simulink model "Copy_9_of_SIMSCAPE_SIM_PROTOTYPE"  (R2024b)
settings: Solver=ode15s  StartTime=0.0  StopTime=T_sim  MaxStep=1e-6  RelTol=1e-6
InitFcn:
  | run param_file.m
values from neighbouring files (symbols this model uses):
  param = struct()    [Copy_of_param_file.m]    (also in param_file.m; param_file_loss_vs_freq.m; param_file_original.m; param_file_turbine.m)
libraries: fl_lib x49, nesl_utility x34, SimscapeFluids_lib x4, eeDcCurrentController x1, ee_lib x1
(part 1 of 2)
settings Model: Creator=user  LastModifiedBy=user
settings SolverCC: MaxConsecutiveMinStep=1000  ZeroCrossAlgorithm=Adaptive
settings DebuggingCC: AlgebraicLoopMsg=none  IgnoredZcDiagnostic=none

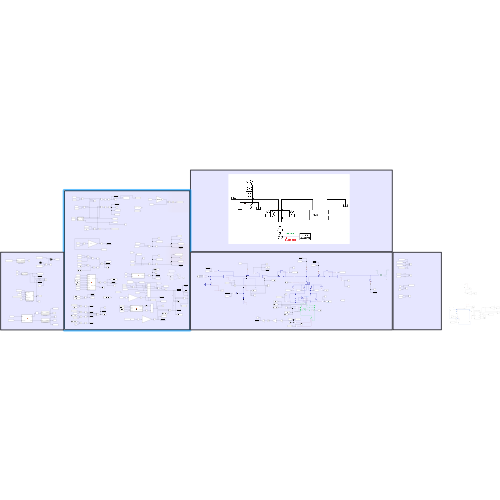
[thumbnail: Simulink's stored preview of the top-level diagram]
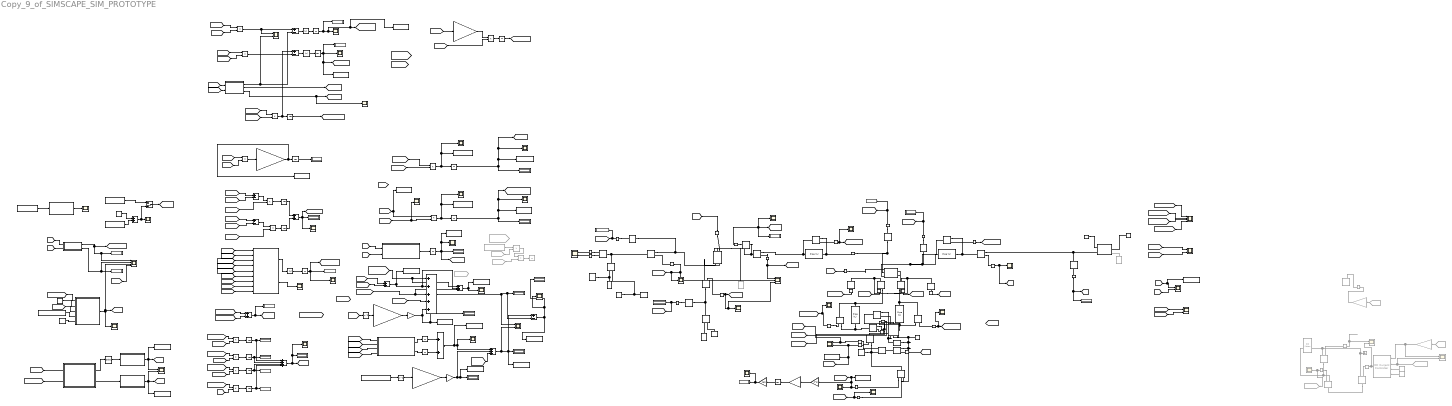
== system Copy_9_of_SIMSCAPE_SIM_PROTOTYPE ==
  note: Control
  note: Energy Calculations
  note: Circuit
  4-Way 2-Position Directional Valve (IL) : SimscapeFluids_lib/Isothermal Liquid/Valves & Orifices/Directional Control Valves/4-Way 2-Position Directional Valve (IL)  open_orifices_pos=fluids.isothermal_liquid.valves_orifices.directional_control_valves.enum.OpenOrifices4Way2Position.PA_BT  open_orifices_neg=fluids.isothermal_liquid.valves_orifices.directional_control_valves.enum.OpenOrifices4Way2Position.PB_AT  area_spec=fluids.isothermal_liquid.valves_orifices.directional_control_valves.enum.directional_valve_area_spec.identical  valve_spec=fluids.isothermal_liquid.valves_orifices.directional_control_valves.enum.directional_valve_spec.linear  del_S_max=param.stroke m  area_max=param.max_Avt m^2  del_S_TLU=[0, .00125, .0025, .00375, .005] m  valve_area_TLU=[1e-10, 1e-05, 4e-05, 6e-05, .0001] m^2  del_S_vol_flow_TLU=[0, .00125, .0025, .00375, .005] m  p_diff_TLU=[-.1, .3, .5, .7] MPa  vol_flow_TLU=[-1e-08, 2.2e-08, 2.8e-08, 3.4e-08; -9e-06, .00015, .0002, .00024; -.00036, .00063, .00081, .00096; -.00054, .00094, .0012, .0014; -.00091, .0016, .002, .0024] m^3/s  p_diff_TLU_const=[-.1, .3, .5, .7] MPa  vol_flow_TLU_const=[-.0009, .0016, .002, .0024] m^3/s  area_const=1e-4 m^2  area_leak=1e-10 m^2  area=inf m^2  Cd=0.64  Re_c=150  smoothing_factor=0.01  pressure_recovery=false  S_max_PA=5e-3 m  del_S_max_PA=0.005 m  area_max_PA=1e-4 m^2  del_S_TLU_PA=[0, .00125, .0025, .00375, .005] m  valve_area_TLU_PA=[1e-10, 1e-05, 4e-05, 6e-05, .0001] m^2  del_S_vol_flow_TLU_PA=[0, .00125, .0025, .00375, .005] m  p_diff_TLU_PA=[-.1, .3, .5, .7] MPa  vol_flow_TLU_PA=[-1e-08, 2.2e-08, 2.8e-08, 3.4e-08; -9e-06, .00015, .0002, .00024; -.00036, .00063, .00081, .00096; -.00054, .00094, .0012, .0014; -.00091, .0016, .002, .0024] m^3/s  area_const_PA=1e-4 m^2  p_diff_TLU_const_PA=[-.1, .3, .5, .7] MPa  vol_flow_TLU_const_PA=[-.0009, .0016, .002, .0024] m^3/s  S_max_PB=-5e-3 m  del_S_max_PB=0.005 m  area_max_PB=1e-4 m^2  del_S_TLU_PB=[0, .00125, .0025, .00375, .005] m  valve_area_TLU_PB=[1e-10, 1e-05, 4e-05, 6e-05, .0001] m^2  del_S_vol_flow_TLU_PB=[0, .00125, .0025, .00375, .005] m  p_diff_TLU_PB=[-.1, .3, .5, .7] MPa  vol_flow_TLU_PB=[-1e-08, 2.2e-08, 2.8e-08, 3.4e-08; -9e-06, .00015, .0002, .00024; -.00036, .00063, .00081, .00096; -.00054, .00094, .0012, .0014; -.00091, .0016, .002, .0024] m^3/s  area_const_PB=1e-4 m^2  p_diff_TLU_const_PB=[-.1, .3, .5, .7] MPa  vol_flow_TLU_const_PB=[-.0009, .0016, .002, .0024] m^3/s  S_max_AT=-5e-3 m  del_S_max_AT=0.005 m  area_max_AT=1e-4 m^2  del_S_TLU_AT=[0, .00125, .0025, .00375, .005] m  valve_area_TLU_AT=[1e-10, 1e-05, 4e-05, 6e-05, .0001] m^2  del_S_vol_flow_TLU_AT=[0, .00125, .0025, .00375, .005] m  p_diff_TLU_AT=[-.1, .3, .5, .7] MPa  vol_flow_TLU_AT=[-1e-08, 2.2e-08, 2.8e-08, 3.4e-08; -9e-06, .00015, .0002, .00024; -.00036, .00063, .00081, .00096; -.00054, .00094, .0012, .0014; -.00091, .0016, .002, .0024] m^3/s  area_const_AT=1e-4 m^2  p_diff_TLU_const_AT=[-.1, .3, .5, .7] MPa  vol_flow_TLU_const_AT=[-.0009, .0016, .002, .0024] m^3/s  S_max_BT=5e-3 m  del_S_max_BT=0.005 m  area_max_BT=1e-4 m^2  del_S_TLU_BT=[0, .00125, .0025, .00375, .005] m  valve_area_TLU_BT=[1e-10, 1e-05, 4e-05, 6e-05, .0001] m^2  del_S_vol_flow_TLU_BT=[0, .00125, .0025, .00375, .005] m  p_diff_TLU_BT=[-.1, .3, .5, .7] MPa  vol_flow_TLU_BT=[-1e-08, 2.2e-08, 2.8e-08, 3.4e-08; -9e-06, .00015, .0002, .00024; -.00036, .00063, .00081, .00096; -.00054, .00094, .0012, .0014; -.00091, .0016, .002, .0024] m^3/s  area_const_BT=1e-4 m^2  p_diff_TLU_const_BT=[-.1, .3, .5, .7] MPa  vol_flow_TLU_const_BT=[-.0009, .0016, .002, .0024] m^3/s
      settings: InternalSimscapePortConfiguration="{\"Bottom\":[{\"id\":\"P\",\"label\":\"P\",\"type\":\"foundation.isothermal_liquid.isothermal_liquid\"},{\"id\":\"T\",\"label\":\"T\",\"type\":\"foundation.isothermal_liquid.isothermal_liquid\"}],\"Left\":[{\"id\":\"S\",\"label\":\"S\",\"type\":\"input\"}],\"Right\":[],\"Top\":[{\"id\":\"A\",\"label\":\"A\",\"type\":\"foundation.isothermal_liquid.isothermal_liquid\"},{\"id\":\"B\",\"label\":\"B\",\"type\":\"foundation.isothermal_liquid.isothermal_liquid\"}]}"
  4-Way 3-Position Directional Valve (IL) : SimscapeFluids_lib/Isothermal Liquid/Valves & Orifices/Directional Control Valves/4-Way 3-Position Directional Valve (IL)  open_orifices_pos=fluids.isothermal_liquid.valves_orifices.directional_control_valves.enum.directional_valve_open_orifices_pos_neg.PA_BT  open_orifices_neu=fluids.isothermal_liquid.valves_orifices.directional_control_valves.enum.directional_valve_open_orifices_neutral.PA_PB_AT_BT  open_orifices_neg=fluids.isothermal_liquid.valves_orifices.directional_control_valves.enum.directional_valve_open_orifices_pos_neg.PB_AT  neutral_assert_action=simscape.enum.assert.action.warn  area_spec=fluids.isothermal_liquid.valves_orifices.directional_control_valves.enum.directional_valve_area_spec.identical  valve_spec=fluids.isothermal_liquid.valves_orifices.directional_control_valves.enum.directional_valve_spec.linear  del_S_max=param.stroke m  area_max=param.max_Avt m^2  del_S_TLU=[0, .00125, .0025, .00375, .005] m  valve_area_TLU=[1e-10, 1e-05, 4e-05, 6e-05, .0001] m^2  del_S_vol_flow_TLU=[0, .00125, .0025, .00375, .005] m  p_diff_TLU=[-.1, .3, .5, .7] MPa  vol_flow_TLU=[-1e-08, 2.2e-08, 2.8e-08, 3.4e-08; -9e-06, .00015, .0002, .00024; -.00036, .00063, .00081, .00096; -.00054, .00094, .0012, .0014; -.00091, .0016, .002, .0024] m^3/s  p_diff_TLU_const=[-.1, .3, .5, .7] MPa  vol_flow_TLU_const=[-.0009, .0016, .002, .0024] m^3/s  area_const=1e-4 m^2  area_leak=1e-10 m^2  area=inf m^2  Cd=0.64  Re_c=150  smoothing_factor=0.01  pressure_recovery=false  S_max_PA=2.5e-3 m  del_S_max_PA=0.005 m  area_max_PA=1e-4 m^2  del_S_TLU_PA=[0, .00125, .0025, .00375, .005] m  valve_area_TLU_PA=[1e-10, 1e-05, 4e-05, 6e-05, .0001] m^2  del_S_vol_flow_TLU_PA=[0, .00125, .0025, .00375, .005] m  p_diff_TLU_PA=[-.1, .3, .5, .7] MPa  vol_flow_TLU_PA=[-1e-08, 2.2e-08, 2.8e-08, 3.4e-08; -9e-06, .00015, .0002, .00024; -.00036, .00063, .00081, .00096; -.00054, .00094, .0012, .0014; -.00091, .0016, .002, .0024] m^3/s  area_const_PA=1e-4 m^2  p_diff_TLU_const_PA=[-.1, .3, .5, .7] MPa  vol_flow_TLU_const_PA=[-.0009, .0016, .002, .0024] m^3/s  S_max_PB=-2.5e-3 m  del_S_max_PB=0.005 m  area_max_PB=1e-4 m^2  del_S_TLU_PB=[0, .00125, .0025, .00375, .005] m  valve_area_TLU_PB=[1e-10, 1e-05, 4e-05, 6e-05, .0001] m^2  del_S_vol_flow_TLU_PB=[0, .00125, .0025, .00375, .005] m  p_diff_TLU_PB=[-.1, .3, .5, .7] MPa  vol_flow_TLU_PB=[-1e-08, 2.2e-08, 2.8e-08, 3.4e-08; -9e-06, .00015, .0002, .00024; -.00036, .00063, .00081, .00096; -.00054, .00094, .0012, .0014; -.00091, .0016, .002, .0024] m^3/s  area_const_PB=1e-4 m^2  p_diff_TLU_const_PB=[-.1, .3, .5, .7] MPa  vol_flow_TLU_const_PB=[-.0009, .0016, .002, .0024] m^3/s  S_max_AB=7.5e-3 m  del_S_max_AB=0.005 m  area_max_AB=1e-4 m^2  del_S_TLU_AB=[0, .00125, .0025, .00375, .005] m  valve_area_TLU_AB=[1e-10, 1e-05, 4e-05, 6e-05, .0001] m^2  del_S_vol_flow_TLU_AB=[0, .00125, .0025, .00375, .005] m  p_diff_TLU_AB=[-.1, .3, .5, .7] MPa  vol_flow_TLU_AB=[-1e-08, 2.2e-08, 2.8e-08, 3.4e-08; -9e-06, .00015, .0002, .00024; -.00036, .00063, .00081, .00096; -.00054, .00094, .0012, .0014; -.00091, .0016, .002, .0024] m^3/s  area_const_AB=1e-4 m^2  p_diff_TLU_const_AB=[-.1, .3, .5, .7] MPa  vol_flow_TLU_const_AB=[-.0009, .0016, .002, .0024] m^3/s  S_max_AT=-2.5e-3 m  del_S_max_AT=0.005 m  area_max_AT=1e-4 m^2  del_S_TLU_AT=[0, .00125, .0025, .00375, .005] m  valve_area_TLU_AT=[1e-10, 1e-05, 4e-05, 6e-05, .0001] m^2  del_S_vol_flow_TLU_AT=[0, .00125, .0025, .00375, .005] m  p_diff_TLU_AT=[-.1, .3, .5, .7] MPa  vol_flow_TLU_AT=[-1e-08, 2.2e-08, 2.8e-08, 3.4e-08; -9e-06, .00015, .0002, .00024; -.00036, .00063, .00081, .00096; -.00054, .00094, .0012, .0014; -.00091, .0016, .002, .0024] m^3/s  area_const_AT=1e-4 m^2  p_diff_TLU_const_AT=[-.1, .3, .5, .7] MPa  vol_flow_TLU_const_AT=[-.0009, .0016, .002, .0024] m^3/s  S_max_BT=2.5e-3 m  del_S_max_BT=0.005 m  area_max_BT=1e-4 m^2  del_S_TLU_BT=[0, .00125, .0025, .00375, .005] m  valve_area_TLU_BT=[1e-10, 1e-05, 4e-05, 6e-05, .0001] m^2  del_S_vol_flow_TLU_BT=[0, .00125, .0025, .00375, .005] m  p_diff_TLU_BT=[-.1, .3, .5, .7] MPa  vol_flow_TLU_BT=[-1e-08, 2.2e-08, 2.8e-08, 3.4e-08; -9e-06, .00015, .0002, .00024; -.00036, .00063, .00081, .00096; -.00054, .00094, .0012, .0014; -.00091, .0016, .002, .0024] m^3/s  area_const_BT=1e-4 m^2  p_diff_TLU_const_BT=[-.1, .3, .5, .7] MPa  vol_flow_TLU_const_BT=[-.0009, .0016, .002, .0024] m^3/s  S_max_PT=0 m  del_S_max_PT=0.005 m  area_max_PT=1e-4 m^2  del_S_TLU_PT=[0, .00125, .0025, .00375, .005] m  valve_area_TLU_PT=[1e-10, 1e-05, 4e-05, 6e-05, .0001] m^2  del_S_vol_flow_TLU_PT=[0, .00125, .0025, .00375, .005] m  p_diff_TLU_PT=[-.1, .3, .5, .7] MPa  vol_flow_TLU_PT=[-1e-08, 2.2e-08, 2.8e-08, 3.4e-08; -9e-06, .00015, .0002, .00024; -.00036, .00063, .00081, .00096; -.00054, .00094, .0012, .0014; -.00091, .0016, .002, .0024] m^3/s
      settings: InternalSimscapePortConfiguration="{\"Bottom\":[{\"id\":\"P\",\"label\":\"P\",\"type\":\"foundation.isothermal_liquid.isothermal_liquid\"},{\"id\":\"T\",\"label\":\"T\",\"type\":\"foundation.isothermal_liquid.isothermal_liquid\"}],\"Left\":[{\"id\":\"S\",\"label\":\"S\",\"type\":\"input\"}],\"Right\":[],\"Top\":[{\"id\":\"A\",\"label\":\"A\",\"type\":\"foundation.isothermal_liquid.isothermal_liquid\"},{\"id\":\"B\",\"label\":\"B\",\"type\":\"foundation.isothermal_liquid.isothermal_liquid\"}]}"
  Abs : Abs  SaturateOnIntegerOverflow=off
  Abs1 : Abs  SaturateOnIntegerOverflow=off
  Abs2 : Abs  SaturateOnIntegerOverflow=off
  Add : Sum  Inputs=+++++
  Add1 : Sum  Inputs=+++
  Add{2..4,6..7} (5 alike) : Sum
  Add5 : Sum  Inputs=++++
  Add8 : Sum  Inputs=+++
  Constant : Constant  Value=param.stroke
  Constant1 : Constant  Value=param.start_final_velocity
  Constant2 : Constant  Value=param.P_H
  Constant3 : Constant  Value=0.75
  Constant4 : Constant  Value=15
  Constant5 : Constant  Value=param.start_final_velocity
  Constant6 : Constant  Value=param.P_M
  Constant7 : Constant  Commented=on  Value=24
  Constant8 : Constant  Commented=on  Value=0
  Constant9 : Constant  Commented=on  Value=param.damping
  Controlled Current Source : fl_lib/Electrical/Electrical Sources/Controlled Current Source  Commented=on
  Controlled Voltage Source : fl_lib/Electrical/Electrical Sources/Controlled Voltage Source  Commented=on
  Current Sensor : fl_lib/Electrical/Electrical Sensors/Current Sensor  Commented=on
  DC Current Controller : eeDcCurrentController/DC Current Controller  Commented=on  Kp=10  Ki=5  Kaw=1  VoltLim=Positive and negative voltage  Ts=-1  Tsd=0.001  ActZC=off
      settings: LibrarySourceBlock=|
      | ee_sl_lib/General Machine
      | Control/DC Current Controller
  DC Motor : ee_lib/Electromechanical/Brushed Motors/DC Motor  Commented=on  field_option=ee.enum.field_option.pm  Rf=100 Ohm  Lf=1 H  Laf=0.15 H  If0=0 A  parameterization=ee.enum.dcparam_option.load_speed  Ra=0.522 Ohm  La=0.625 mH  emf_or_torque=ee.enum.emf_or_torque.ki  Kv=1/param.Kv V*s/rad  Ki=param.Kt N*m/A  T_stall=7480 m*mN  w_max=3120 rpm  w_rated=2510 rpm  P_rated=147 W  V_rated=36 V  lam_param=ee.enum.lam_param.current  i_noload=348 mA  V_i_noload=36 V  J=0 kg*m^2  lam=0 N*m*s/rad  speed0=param.start_final_velocity rad/s  t_fault_armature=1 s  t_fault_field=1 s  fault_action=simscape.enum.assert.action.none  alpha=3.93e-3 1/K  Tmeas=25 degC  thermal_mass=100 J/K  initial_temperature=25 degC
  Display{,1..16} (17 alike) : Display
  Double-Acting Actuator (IL)1 : SimscapeFluids_lib/Isothermal Liquid/Actuators/Double-Acting Actuator (IL)  single_fluid=true  mech_orientation=foundation.enum.MechOrientationTranslational.Positive  piston_area_A=param.Acap m^2  piston_area_B=4e-4 m^2  stroke=param.V1_0/param.Acap m  dead_volume_A=1e-5 m^3  dead_volume_B=1e-5 m^3  pressure_spec=foundation.enum.pressure_spec.atmospheric  environment_pressure=0.101325 MPa  hardstop_model=simscape.enum.hardstop.smooth  stiff_coeff=1e10 N/m  damping_coeff=150 N*s/m  transition=0.1 mm  coeff_rest=0.7  v_tol=0.001 m/s  f_tol=0.001 N  cushion_A_spec=false  area_plunger_A=1e-4 m^2  length_plunger_A=1e-3 m  area_cushion_orifice_A=1e-6 m^2  area_leak_plunger_A=1e-7 m^2  p_crack_differential_A=0.01 MPa  press_max_differential_A=0.1 MPa  check_valve_area_max_A=1e-4 m^2  check_valve_area_leak_A=1e-10 m^2  smoothing_factor_A=0.01  cushion_B_spec=false  area_plunger_B=1e-4 m^2  length_plunger_B=1e-3 m  area_cushion_orifice_B=1e-6 m^2  area_leak_plunger_B=1e-7 m^2  p_crack_differential_B=0.01 MPa  press_max_differential_B=0.1 MPa  check_valve_area_max_B=1e-4 m^2  check_valve_area_leak_B=1e-10 m^2  smoothing_factor_B=0.01  friction_spec=false  breakaway_Coulomb_ratio=1.2  breakaway_velocity=0.1 m/s  preload_force=20 N  Coulomb_coeff=1e-6 N/Pa  viscous_coeff=100 N*s/m  leakage_spec=false  clearance=1e-4 m  piston_length=0.01 m  displacement_spec=foundation.enum.DisplacementSpec.Calculate  x0=param.V1_0/param.Acap m  dynamic_compressibility=true  p0_A=param.P_initial+param.P_T Pa  p0_B=param.P_T Pa
      settings: InternalSimscapePortConfiguration="{\"Bottom\":[],\"Left\":[{\"id\":\"C\",\"label\":\"C\",\"type\":\"foundation.mechanical.translational.translational\"},{\"id\":\"A\",\"label\":\"A\",\"type\":\"foundation.isothermal_liquid.isothermal_liquid\"}],\"Right\":[{\"id\":\"p_out\",\"label\":\"p\",\"type\":\"output\"},{\"id\":\"R\",\"label\":\"R\",\"type\":\"foundation.mechanical.translational.translational\"},{\"id\":\"B\",\"label\":\"B\",\"type\":\"foundation.isothermal_liquid.isothermal_liquid\"}],\"Top\":[]}"
  Dynamics of Orifice 3 : Subsystem
  Electric Torque Controller1 : MATLAB Function  TreatAsAtomicUnit=on
  Electrical Reference : fl_lib/Electrical/Electrical Elements/Electrical Reference  Commented=on
  Energy In : Display
  Energy Out : Display
  Fixed-Displacement Motor (IL) : SimscapeFluids_lib/Isothermal Liquid/Pumps & Motors/Fixed-Displacement Motor (IL)  leakage_friction_spec=fluids.isothermal_liquid.pumps_motors.enum.MotorLossSpec.Analytical  displacement=param.D m^3/rev  omega_nominal=1000 rpm  p_nominal=21 MPa  vol_eff_nominal=param.pump_vol_eff  mech_eff_nominal=param.pump_mech_eff  no_load_torque=0 N*m  p_diff_eff_TLU=[.1, 1, 2] MPa  omega_eff_TLU=[250, 500, 1000, 2000, 3000, 4000] rpm  vol_eff_TLU=[.816, .908, .954, .977, .981, .984; .325, .663, .831, .916, .925, .946; .137, .568, .78, .892, .893, .91]  mech_eff_TLU=[.996, .996, .996, .996, .996, .996; .988, .989, .989, .989, .989, .99; .981, .981, .982, .982, .983, .984]  p_diff_loss_TLU=[.1, 1, 2] MPa  omega_loss_TLU=[250, 500, 1000, 2000, 3000, 4000] rpm  vol_loss_TLU=1e-3 * [.023, .023, .023, .023, .0285, .032; .0844, .0842, .0845, .084, .1125, .108; .1079, .108, .11, .108, .1605, .18] m^3/s  mech_loss_TLU=[.002, .002, .002, .002, .002, .002; .0607, .0556, .0556, .0556, .0556, .0505; .1937, .1937, .1833, .1833, .1729, .1626] N*m  q_shaft_TLU=[.125, .25, .5, 1, 1.5, 2] * 1e-3 m^3/s  p_diff_shaft_TLU=[.1, 1, 2] MPa  torque_shaft_TLU=[.47, 4.72, 9.35; .47, 4.7, 9.36; .47, 4.7, 9.4; .47, 4.7, 9.41; .47, 4.7, 9.46; .47, 4.68, 9.5] N*m  omega_shaft_TLU=[205, 80, 35; 455, 330, 285; 955, 831, 780; 1950, 1830, 1780; 2940, 2775, 2680; 3940, 3780, 3640] rpm  vol_eff_min=1e-3  vol_eff_max=1  mech_eff_min=1e-3  mech_eff_max=1  pressure_threshold=1e-3 MPa  omega_threshold=100 rpm  supplied_range_check=simscape.enum.assert.action.none  motor_mode_check=simscape.enum.assert.action.none  pressure_check=simscape.enum.assert.action.none  p_min_valid=0.101325 MPa
      settings: InternalSimscapePortConfiguration="{\"Bottom\":[{\"id\":\"B\",\"label\":\"B\",\"type\":\"foundation.isothermal_liquid.isothermal_liquid\"}],\"Left\":[],\"Right\":[{\"id\":\"R\",\"label\":\"R\",\"type\":\"foundation.mechanical.rotational.rotational\"},{\"id\":\"C\",\"label\":\"C\",\"type\":\"foundation.mechanical.rotational.rotational\"}],\"Top\":[{\"id\":\"A\",\"label\":\"A\",\"type\":\"foundation.isothermal_liquid.isothermal_liquid\"}]}"
  Flow Rate Sensor (IL){,1..7} (8 alike) : fl_lib/Isothermal Liquid/Sensors/Flow Rate Sensor (IL)  sensor_type=foundation.enum.mass_volumetric_sensor.volumetric
      settings: InternalSimscapePortConfiguration="{\"Bottom\":[],\"Left\":[{\"id\":\"A\",\"label\":\"A\",\"type\":\"foundation.isothermal_liquid.isothermal_liquid\"}],\"Right\":[{\"id\":\"B\",\"label\":\"B\",\"type\":\"foundation.isothermal_liquid.isothermal_liquid\"},{\"id\":\"V\",\"label\":\"V\",\"type\":\"output\"}],\"Top\":[]}"
  For the big Valve : Subsystem
  For the small Valve : Subsystem
  From11 : From  Commented=on  GotoTag=T_elec
  From46 : From  Commented=on  GotoTag=Current_arm
  From54 : From  Commented=on  GotoTag=T_elec
  From62 : From  Commented=on  GotoTag=omega
  From63 : From  Commented=on  GotoTag=omega
  From77 : From  Commented=on  GotoTag=elec_motor_losses
  From79 : From  Commented=on  GotoTag=Regen_Elec
  Gain : Gain  Commented=on  Gain=1/(param.Kt)
  Gain1 : Gain  Gain=param.J_elec+param.J_hyd
  Gain10 : Gain  Gain=param.damping
  Gain2 : Gain  Gain=0.5
  Gain3 : Gain  Gain=param.D
  Gain4 : Gain  Gain=param.J_elec+param.J_hyd
  Gain5 : Gain  Gain=0.5
  Gain6 : Gain  Gain=param.J_elec+param.J_hyd
  Gain7 : Gain  Commented=on  Gain=1/(param.Kt)
  Gain8 : Gain  Gain=2*pi
  Gain9 : Gain  Gain=1e6
  Goto30 : Goto  Commented=on  GotoTag=Current_arm
  Hydraulic Motor Inertia : fl_lib/Mechanical/Rotational Elements/Inertia  inertia=(param.J_hyd+param.J_elec) kg*m^2  num_ports=foundation.enum.numPorts2.one  w_specify=on  w_priority=High  w=param.start_final_velocity rad/s  w_nominal_specify=off  w_nominal_value=1  w_nominal_unit=rad/s  t_specify=off  t_priority=None  t=0 N*m  t_nominal_specify=off  t_nominal_value=1  t_nominal_unit=N*m
  Ideal Rotational Motion Sensor1 : fl_lib/Mechanical/Mechanical Sensors/Ideal Rotational Motion Sensor  reference=foundation.enum.MeasurementReference.difference  acceleration_port=true  velocity_port=true  position_port=false  wrap_angle=false  offset=0 rad
      settings: InternalSimscapePortConfiguration="{\"Bottom\":[],\"Left\":[{\"id\":\"R\",\"label\":\"R\",\"type\":\"foundation.mechanical.rotational.rotational\"}],\"Right\":[{\"id\":\"C\",\"label\":\"C\",\"type\":\"foundation.mechanical.rotational.rotational\"},{\"id\":\"alpha\",\"label\":\"α\",\"type\":\"output\"},{\"id\":\"W\",\"label\":\"W\",\"type\":\"output\"}],\"Top\":[]}"
  Ideal Torque Sensor : fl_lib/Mechanical/Mechanical Sensors/Ideal Torque Sensor
  Ideal Torque Sensor1 : fl_lib/Mechanical/Mechanical Sensors/Ideal Torque Sensor
  Ideal Torque Source : fl_lib/Mechanical/Mechanical Sources/Ideal Torque Source
  Initial Kinetic Energy : Display
  Integrator{,1..10,12,14..17,20..21} (18 alike) : Integrator
  Integrator13 : Integrator  Commented=on
  Isothermal Liquid Properties (IL) : fl_lib/Isothermal Liquid/Utilities/Isothermal Liquid Properties (IL)  rho_L_atm=param.rho kg/m^3  bulk_modulus_model=foundation.enum.bulk_modulus_model.const  beta_gain=6  beta_L_atm=param.beta Pa  nu_atm=1.0034e-6 m^2/s  p_atm=0.101325 MPa  p_min=1 Pa  properties_range_check=simscape.enum.assert.action.error  air_fraction=0.005  polytropic_index=1.0  rho_g_atm=1.225 kg/m^3  air_dissolution_model=false  p_crit=1 MPa
  Liquid Properties Sensor (IL) : fl_lib/Isothermal Liquid/Sensors/Liquid Properties Sensor (IL)  density_measure=false  bulk_modulus_measure=true  entrained_air_measure=true
      settings: InternalSimscapePortConfiguration="{\"Bottom\":[],\"Left\":[{\"id\":\"A\",\"label\":\"A\",\"type\":\"foundation.isothermal_liquid.isothermal_liquid\"}],\"Right\":[{\"id\":\"beta\",\"label\":\"beta\",\"type\":\"output\"},{\"id\":\"theta\",\"label\":\"theta\",\"type\":\"output\"}],\"Top\":[]}"
  MATLAB Function1 : MATLAB Function  TreatAsAtomicUnit=on
  MATLAB Function2 : MATLAB Function  TreatAsAtomicUnit=on
  MATLAB Function3 : MATLAB Function  TreatAsAtomicUnit=on
  MATLAB Function4 : MATLAB Function  TreatAsAtomicUnit=on
  MATLAB Function6 : MATLAB Function  TreatAsAtomicUnit=on
  Manual Switch : ManualSwitch  CurrentSetting=0
  Mechanical Rotational Reference2 : fl_lib/Mechanical/Rotational Elements/Mechanical Rotational Reference
  Mechanical Translational Reference2 : fl_lib/Mechanical/Translational Elements/Mechanical Translational Reference
  Mechanical Translational Reference3 : fl_lib/Mechanical/Translational Elements/Mechanical Translational Reference
  Mechanical Energy : Display
  PS Constant : fl_lib/Physical Signals/Sources/PS Constant  constant=param.P_H Pa
  PS Constant1 : fl_lib/Physical Signals/Sources/PS Constant  constant=param.P_M Pa
  PS-Simulink Converter : nesl_utility/PS-Simulink Converter  PhysicalDomain=network_engine_domain  SubClassName=ps_output  LeftPortType=input  RightPortType=output  PseudoPeriodic=off  Frequencies=[]  VectorFormat=inherit  Unit=m^3/s  AffineConversion=off
  PS-Simulink Converter1 : nesl_utility/PS-Simulink Converter  PhysicalDomain=network_engine_domain  SubClassName=ps_output  LeftPortType=input  RightPortType=output  PseudoPeriodic=off  Frequencies=[]  VectorFormat=inherit  Unit=rad/s  AffineConversion=off
  PS-Simulink Converter10 : nesl_utility/PS-Simulink Converter  PhysicalDomain=network_engine_domain  SubClassName=ps_output  LeftPortType=input  RightPortType=output  PseudoPeriodic=off  Frequencies=[]  VectorFormat=inherit  Unit=Pa  AffineConversion=off
  PS-Simulink Converter11 : nesl_utility/PS-Simulink Converter  PhysicalDomain=network_engine_domain  SubClassName=ps_output  LeftPortType=input  RightPortType=output  PseudoPeriodic=off  Frequencies=[]  VectorFormat=inherit  Unit=m^3/s  AffineConversion=off
  PS-Simulink Converter12 : nesl_utility/PS-Simulink Converter  PhysicalDomain=network_engine_domain  SubClassName=ps_output  LeftPortType=input  RightPortType=output  PseudoPeriodic=off  Frequencies=[]  VectorFormat=inherit  Unit=m^3/s  AffineConversion=off
  PS-Simulink Converter{3..9,13..19,21,23..27} (20 alike) : nesl_utility/PS-Simulink Converter  PhysicalDomain=network_engine_domain  SubClassName=ps_output  LeftPortType=input  RightPortType=output  PseudoPeriodic=off  Frequencies=[]  VectorFormat=inherit  Unit=inherit  AffineConversion=off
  PS-Simulink Converter2 : nesl_utility/PS-Simulink Converter  PhysicalDomain=network_engine_domain  SubClassName=ps_output  LeftPortType=input  RightPortType=output  PseudoPeriodic=off  Frequencies=[]  VectorFormat=inherit  Unit=Pa  AffineConversion=off
  PS-Simulink Converter20 : nesl_utility/PS-Simulink Converter  Commented=on  PhysicalDomain=network_engine_domain  SubClassName=ps_output  LeftPortType=input  RightPortType=output  PseudoPeriodic=off  Frequencies=[]  VectorFormat=inherit  Unit=inherit  AffineConversion=off
  PS-Simulink Converter22 : nesl_utility/PS-Simulink Converter  Commented=on  PhysicalDomain=network_engine_domain  SubClassName=ps_output  LeftPortType=input  RightPortType=output  PseudoPeriodic=off  Frequencies=[]  VectorFormat=inherit  Unit=inherit  AffineConversion=off
  Pipe (IL)2 : fl_lib/Isothermal Liquid/Elements/Pipe (IL)  length=0.2 m  area=0.25*pi*(param.D_hose)^2 mm^2  Dh=param.D_hose mm  length_add=0.5 m  roughness=15e-6 m  Re_lam=2000  Re_tur=4000  shape_factor=64  dynamic_compressibility=true  inertia=false  p0=param.P_initial+param.P_T Pa  mdot0=0 kg/s
      settings: InternalSimscapePortConfiguration="{\"Bottom\":[],\"Left\":[{\"id\":\"A\",\"label\":\"A\",\"type\":\"foundation.isothermal_liquid.isothermal_liquid\"}],\"Right\":[{\"id\":\"B\",\"label\":\"B\",\"type\":\"foundation.isothermal_liquid.isothermal_liquid\"}],\"Top\":[]}"
  Pipe (IL)3 : fl_lib/Isothermal Liquid/Elements/Pipe (IL)  length=0.2 m  area=0.25*pi*(param.D_hose)^2 mm^2  Dh=param.D_hose mm  length_add=0.5 m  roughness=15e-6 m  Re_lam=2000  Re_tur=4000  shape_factor=64  dynamic_compressibility=true  inertia=false  p0=param.P_initial+param.P_T Pa  mdot0=0 kg/s
      settings: InternalSimscapePortConfiguration="{\"Bottom\":[],\"Left\":[{\"id\":\"A\",\"label\":\"A\",\"type\":\"foundation.isothermal_liquid.isothermal_liquid\"}],\"Right\":[{\"id\":\"B\",\"label\":\"B\",\"type\":\"foundation.isothermal_liquid.isothermal_liquid\"}],\"Top\":[]}"
  Pipe (IL)4 : fl_lib/Isothermal Liquid/Elements/Pipe (IL)  length=0.2 m  area=0.25*pi*(param.D_hose)^2 mm^2  Dh=param.D_hose mm  length_add=0.5 m  roughness=15e-6 m  Re_lam=2000  Re_tur=4000  shape_factor=64  dynamic_compressibility=true  inertia=false  p0=param.P_initial+param.P_T Pa  mdot0=0 kg/s
      settings: InternalSimscapePortConfiguration="{\"Bottom\":[],\"Left\":[{\"id\":\"A\",\"label\":\"A\",\"type\":\"foundation.isothermal_liquid.isothermal_liquid\"}],\"Right\":[{\"id\":\"B\",\"label\":\"B\",\"type\":\"foundation.isothermal_liquid.isothermal_liquid\"}],\"Top\":[]}"
  Pipe (IL)5 : fl_lib/Isothermal Liquid/Elements/Pipe (IL)  length=1 m  area=0.25*pi*(param.D_hose)^2 mm^2  Dh=param.D_hose mm  length_add=0.5 m  roughness=15e-6 m  Re_lam=2000  Re_tur=4000  shape_factor=64  dynamic_compressibility=true  inertia=false  p0=param.P_initial+param.P_T Pa  mdot0=0 kg/s
      settings: InternalSimscapePortConfiguration="{\"Bottom\":[],\"Left\":[{\"id\":\"A\",\"label\":\"A\",\"type\":\"foundation.isothermal_liquid.isothermal_liquid\"}],\"Right\":[{\"id\":\"B\",\"label\":\"B\",\"type\":\"foundation.isothermal_liquid.isothermal_liquid\"}],\"Top\":[]}"
  Pressure Sensor (IL){,1..5,10..11} (8 alike) : fl_lib/Isothermal Liquid/Sensors/Pressure Sensor (IL)  pressure_measure=foundation.enum.pressure_measure.gauge
      settings: InternalSimscapePortConfiguration="{\"Bottom\":[],\"Left\":[{\"id\":\"A\",\"label\":\"A\",\"type\":\"foundation.isothermal_liquid.isothermal_liquid\"}],\"Right\":[{\"id\":\"Pg\",\"label\":\"Pg\",\"type\":\"output\"}],\"Top\":[]}"
  Pressure Sensor (IL){6..9,12} (5 alike) : fl_lib/Isothermal Liquid/Sensors/Pressure Sensor (IL)  pressure_measure=foundation.enum.pressure_measure.difference
      settings: InternalSimscapePortConfiguration="{\"Bottom\":[],\"Left\":[{\"id\":\"A\",\"label\":\"A\",\"type\":\"foundation.isothermal_liquid.isothermal_liquid\"}],\"Right\":[{\"id\":\"B\",\"label\":\"B\",\"type\":\"foundation.isothermal_liquid.isothermal_liquid\"},{\"id\":\"P\",\"label\":\"P\",\"type\":\"output\"}],\"Top\":[]}"
  Pressure Source (IL)1 : fl_lib/Isothermal Liquid/Sources/Pressure Source (IL)  source_type=foundation.enum.constant_controlled.controlled  pressure_differential=0 MPa
      settings: InternalSimscapePortConfiguration="{\"Bottom\":[],\"Left\":[{\"id\":\"A\",\"label\":\"A\",\"type\":\"foundation.isothermal_liquid.isothermal_liquid\"},{\"id\":\"P\",\"label\":\"P\",\"type\":\"input\"}],\"Right\":[{\"id\":\"B\",\"label\":\"B\",\"type\":\"foundation.isothermal_liquid.isothermal_liquid\"}],\"Top\":[]}"
  Pressure Source (IL)2 : fl_lib/Isothermal Liquid/Sources/Pressure Source (IL)  source_type=foundation.enum.constant_controlled.controlled  pressure_differential=0 MPa
      settings: InternalSimscapePortConfiguration="{\"Bottom\":[],\"Left\":[{\"id\":\"A\",\"label\":\"A\",\"type\":\"foundation.isothermal_liquid.isothermal_liquid\"},{\"id\":\"P\",\"label\":\"P\",\"type\":\"input\"}],\"Right\":[{\"id\":\"B\",\"label\":\"B\",\"type\":\"foundation.isothermal_liquid.isothermal_liquid\"}],\"Top\":[]}"
  Product{,1..10,13..14} (13 alike) : Product
  Product11 : Product  Commented=on
  Product12 : Product  Commented=on
  Pulse Generator : DiscretePulseGenerator  PulseType=Time based  Amplitude=param.P_H-param.P_M  Period=param.T_period  PulseWidth=50  PhaseDelay=param.delay
  Regen : Display
  Regen1 : Display
  Reservoir (IL)1 : fl_lib/Isothermal Liquid/Elements/Reservoir (IL)  reservoir_type=foundation.enum.constant_controlled.constant  pressure_spec=foundation.enum.pressure_spec.atmospheric  reservoir_pressure=0.101325 MPa
  Reservoir (IL)5 : fl_lib/Isothermal Liquid/Elements/Reservoir (IL)  reservoir_type=foundation.enum.constant_controlled.constant  pressure_spec=foundation.enum.pressure_spec.atmospheric  reservoir_pressure=0.101325 MPa
  Reservoir (IL)7 : fl_lib/Isothermal Liquid/Elements/Reservoir (IL)  Commented=on  reservoir_type=foundation.enum.constant_controlled.constant  pressure_spec=foundation.enum.pressure_spec.atmospheric  reservoir_pressure=0.101325 MPa
  Reservoir (IL)8 : fl_lib/Isothermal Liquid/Elements/Reservoir (IL)  Commented=on  reservoir_type=foundation.enum.constant_controlled.constant  pressure_spec=foundation.enum.pressure_spec.atmospheric  reservoir_pressure=0.101325 MPa
  Rotational Damper : fl_lib/Mechanical/Rotational Elements/Rotational Damper  D=param.damping N*m*s/rad  w_specify=on  w_priority=None  w=param.start_final_velocity rad/s  w_nominal_specify=off  w_nominal_value=1  w_nominal_unit=rad/s  t_specify=off  t_priority=None  t=0 N*m  t_nominal_specify=off  t_nominal_value=1  t_nominal_unit=N*m
  Scope{,1,4,6,8,16,23,27,41} (9 alike) : Scope  NumInputPorts=2
  Scope{2..3,7,10..15,17..21,26,28..34,36..40,42} (28 alike) : Scope
  Scope22 : Scope  Commented=on
  Scope24 : Scope  Commented=on  NumInputPorts=2
  Scope25 : Scope  Commented=on  NumInputPorts=2
  Scope35 : Scope  NumInputPorts=3
  Scope5 : Scope  NumInputPorts=4
  Scope9 : Scope  NumInputPorts=4
  Simulink-PS Converter : nesl_utility/Simulink-PS Converter  PhysicalDomain=network_engine_domain  SubClassName=ps_input  LeftPortType=input  RightPortType=output  PseudoPeriodic=off  Frequencies=[]  NoiseDistribution=none  NoiseParameters=[]  Unit=1  AffineConversion=off  FilteringAndDerivatives=provide  SimscapeFilterOrder=1  InputFilterTimeConstant=0.001  UdotUserProvided=0
  Simulink-PS Converter1 : nesl_utility/Simulink-PS Converter  PhysicalDomain=network_engine_domain  SubClassName=ps_input  LeftPortType=input  RightPortType=output  PseudoPeriodic=off  Frequencies=[]  NoiseDistribution=none  NoiseParameters=[]  Unit=1  AffineConversion=off  FilteringAndDerivatives=provide  SimscapeFilterOrder=1  InputFilterTimeConstant=0.001  UdotUserProvided=0
  Simulink-PS Converter2 : nesl_utility/Simulink-PS Converter  Commented=on  PhysicalDomain=network_engine_domain  SubClassName=ps_input  LeftPortType=input  RightPortType=output  PseudoPeriodic=off  Frequencies=[]  NoiseDistribution=none  NoiseParameters=[]  Unit=1  AffineConversion=off  FilteringAndDerivatives=provide  SimscapeFilterOrder=1  InputFilterTimeConstant=0.001  UdotUserProvided=0
  Simulink-PS Converter3 : nesl_utility/Simulink-PS Converter  Commented=on  PhysicalDomain=network_engine_domain  SubClassName=ps_input  LeftPortType=input  RightPortType=output  PseudoPeriodic=off  Frequencies=[]  NoiseDistribution=none  NoiseParameters=[]  Unit=1  AffineConversion=off  FilteringAndDerivatives=provide  SimscapeFilterOrder=1  InputFilterTimeConstant=0.001  UdotUserProvided=0
  Simulink-PS Converter4 : nesl_utility/Simulink-PS Converter  PhysicalDomain=network_engine_domain  SubClassName=ps_input  LeftPortType=input  RightPortType=output  PseudoPeriodic=off  Frequencies=[]  NoiseDistribution=none  NoiseParameters=[]  Unit=1  AffineConversion=off  FilteringAndDerivatives=provide  SimscapeFilterOrder=1  InputFilterTimeConstant=0.001  UdotUserProvided=0
  Solver Configuration1 : nesl_utility/Solver Configuration  PhysicalDomain=network_engine_domain  SubClassName=solver  LeftPortType=input  RightPortType=generic  Tones=[]  Harmonics=[]  SimulateNoise=off  Profile=off  UseLocalSampling=off  EnableSwitchedLinearOptims=on  FrequencyDomain=off  UseCCode=off  RelTol=0.001  AbsTol=0.001  MinStep=1e-09  ToWorkspace=off  RevertToSquareIcSolve=off  NumHomotopyIterations=100  PhasorMode=off  PhasorModeNumHarmonics=1  ConsistencySolver=NEWTON_XTOL_AFTER_FTOL  IndexReductionMethod=DerivativeReplacement  DoDC=off  ResidualTolerance=1e-09  ConsistencyTolSource=GLOBAL  ConsistencyAbsTol=0.001  ConsistencyRelTol=0.001  ConsistencyTolFactor=0.001  UseLocalSolver=off  LocalSolverChoice=NE_BACKWARD_EULER_ADVANCER  ResolveIndetEquations=on  FunctionEvalNumThread=1  LocalSolverSampleTime=0.001  DoFixedCost=off  MaxNonlinIter=3  MaxModeIter=2  ComputeImpulses=off  ImpulseIterations=2  LinearAlgebra=auto  LinearAlgebraNumThread=0  EquationFormulation=NE_TIME_EF  DelaysMemoryBudget=1024  AutomaticFiltering=on  FilteringTimeConstant=0.001  PartitionStorageMethod=AS_NEEDED  PartitionMemoryBudget=1024  PartitionMethod=ROBUST  MultibodyUseLocalSolver=off  MultibodyLocalSolverChoice=ODE1  MultibodyLocalSolverSampleTime=0.001
  Square1 : Math  Operator=square
  Square2 : Math  Operator=square
  Stored : Display
  Subsystem : Subsystem
  Subtract{,1..4} (5 alike) : Sum  Inputs=+-
  Throttling Loss Big Valve : Display
  Throttling Loss Small Valve1 : Display
  Throttling Total : Display
  To Workspace : ToWorkspace  VariableName=Stored  SaveFormat=Timeseries  SampleTime=-1
  To Workspace1 : ToWorkspace  VariableName=Regen_Mech  SaveFormat=Timeseries  SampleTime=-1
  To Workspace10 : ToWorkspace  VariableName=Hyd_Energy_In  SaveFormat=Timeseries  SampleTime=-1
  To Workspace11 : ToWorkspace  VariableName=Work_Out  SaveFormat=Timeseries  SampleTime=-1
  To Workspace12 : ToWorkspace  VariableName=Regen_Elec  SaveFormat=Timeseries  SampleTime=-1
  To Workspace13 : ToWorkspace  VariableName=Regen_power_Elec  SaveFormat=Timeseries  SampleTime=-1
  To Workspace14 : ToWorkspace  VariableName=Throttling_Losses  SaveFormat=Timeseries  SampleTime=-1
  To Workspace15 : ToWorkspace  VariableName=T_elec_2  SaveFormat=Timeseries  SampleTime=-1
  To Workspace16 : ToWorkspace  VariableName=Pump_Losses  SaveFormat=Timeseries  SampleTime=-1
  To Workspace17 : ToWorkspace  VariableName=elec_motor_losses  SaveFormat=Timeseries  SampleTime=-1
  To Workspace18 : ToWorkspace  VariableName=S_big  SaveFormat=Timeseries  SampleTime=-1
  To Workspace19 : ToWorkspace  VariableName=S_small  SaveFormat=Timeseries  SampleTime=-1
  To Workspace2 : ToWorkspace  VariableName=KE  SaveFormat=Timeseries  SampleTime=-1
  To Workspace20 : ToWorkspace  VariableName=Losses  SaveFormat=Timeseries  SampleTime=-1
  To Workspace3 : ToWorkspace  VariableName=P1  SaveFormat=Timeseries  SampleTime=-1
  To Workspace4 : ToWorkspace  VariableName=T_elec  SaveFormat=Timeseries  SampleTime=-1
  To Workspace5 : ToWorkspace  VariableName=omega  SaveFormat=Timeseries  SampleTime=-1
  To Workspace6 : ToWorkspace  VariableName=Regen_power_Mech  SaveFormat=Timeseries  SampleTime=-1
  To Workspace7 : ToWorkspace  VariableName=mech_power  SaveFormat=Timeseries  SampleTime=-1
  To Workspace8 : ToWorkspace  VariableName=Energy_In  SaveFormat=Timeseries  SampleTime=-1
  To Workspace9 : ToWorkspace  VariableName=Initial_kinetic  SaveFormat=Timeseries  SampleTime=-1
  Transport Delay2 : TransportDelay  DelayTime=10e-3  InitialOutput=param.initial_stroke  BufferSize=1024*105
  Voltage Sensor : fl_lib/Electrical/Electrical Sensors/Voltage Sensor  Commented=on
  Work Out Actual1 : Display
  wires:
  [P1] -> Subsystem/1(P1)
  Subsystem/1(Control_Signal) -> [Control_Signal], Scope5/1, Display1/1  "Control Signal"
  [Pdes] -> Subsystem/2(Pdes)
  PS-Simulink Converter3/1 -> [P1], Display2/1
  Subsystem/2(delP) -> Scope5/2, Display4/1  "delP"
  PS-Simulink Converter1/1 -> Scope2/1, To Workspace5/1, [omega], Gain8/1
  PS-Simulink Converter5/1 -> Scope6/1  "Entrained Air"
  PS-Simulink Converter6/1 -> Scope6/2  "Bulk Modulus"
  PS-Simulink Converter/1 -> [Qout], Scope7/1
  Constant/1 -> Dynamics of Orifice 3/1(Stroke)
  Dynamics of Orifice 3/1(Spool Opening) -> Scope10/1
  PS-Simulink Converter9/1 -> Scope35/1, [Q_A_big]
  PS-Simulink Converter4/1 -> Scope35/2, Scope34/1, [Q_P_big]
  PS-Simulink Converter8/1 -> Display5/1, Scope13/1, [P_A_big]
  [omega] -> Scope4/2, Product2/2
  Product2/1 -> Scope11/1, To Workspace6/1, Integrator7/1
  MATLAB Function1/1(Power_out) -> Integrator17/1
  Integrator17/1 -> [Work_Out], To Workspace11/1, Scope20/1, Work Out Actual1/1
  [P1] -> MATLAB Function1/1(P1)
  [Qout] -> MATLAB Function1/2(Qout)
  PS-Simulink Converter10/1 -> [P_P_small]
  PS-Simulink Converter2/1 -> [P_T_small]
  PS-Simulink Converter12/1 -> [Q_T_small]
  PS-Simulink Converter11/1 -> [Q_P_small]
  Constant5/1 -> Electric Torque Controller1/4(start_final_velocity)
  [omega] -> Electric Torque Controller1/3(omega)
  Constant4/1 -> Electric Torque Controller1/2(Kp)
  [Control_Signal] -> Electric Torque Controller1/1(Control_Signal)
  Electric Torque Controller1/1(T_elec) -> Scope5/3, [T_elec], Scope3/1  "T_elec"
  PS-Simulink Converter13/1 -> Scope35/3, Scope14/1, [Q_T_big]
  PS-Simulink Converter7/1 -> Display/1, [P_P_big]
  Integrator7/1 -> Scope19/1, [Regen_Mech], To Workspace1/1, Regen/1  "Regen"
  From11/1 -> Gain/1
  Transport Delay2/1 -> For the big Valve/1(Stroke)
  [Control_Signal] -> MATLAB Function2/2(Control_signal)
  [Pdes] -> MATLAB Function2/1(Pdes)
  [S_big] -> Simulink-PS Converter/1
  [S_small] -> Simulink-PS Converter1/1
  MATLAB Function2/1(S_big) -> Transport Delay2/1
  MATLAB Function2/2(S_small) -> For the small Valve/1(Stroke)
  For the big Valve/1(Spool Opening) -> To Workspace18/1, Scope1/1, [S_big]
  For the small Valve/1(Spool Opening) -> Scope1/2, To Workspace19/1, [S_small]
  Constant3/1 -> Electric Torque Controller1/5(T_elec_max)
  Pulse Generator/1 -> Add2/1
  Constant6/1 -> Add2/2
  Add2/1 -> Manual Switch/2, Scope12/1
  Constant2/1 -> Manual Switch/1
  Manual Switch/1 -> [Pdes]
  PS-Simulink Converter14/1 -> [P_T_big], Display3/1
  [P_P_big] -> Subtract/1
  [P_A_big] -> Subtract/2
  [Q_P_big] -> Product/2
  Subtract/1 -> Product/1
  Product/1 -> Integrator1/1
  Integrator1/1 -> Add4/1
  Subtract1/1 -> Product3/1
  [Q_T_big] -> Product3/2
  Product3/1 -> Integrator3/1
  Integrator3/1 -> Add4/2
  Add4/1 -> Scope30/1, [Throttling_1], Throttling Loss Big Valve/1
  [Qout] -> Scope9/1  "Qout"
  [Q_A_big] -> Scope9/2  "Q_A_big"
  [Q_P_small] -> Scope9/3  "Q_P_small"
  [Q_T_small] -> Scope9/4  "Q_T_small"
  PS-Simulink Converter15/1 -> Scope36/1, [Pdrop_hose_1]
  PS-Simulink Converter16/1 -> Scope33/1, [Pdrop_hose_2]
  PS-Simulink Converter17/1 -> Scope40/1, [Pdrop_hose_3]
  PS-Simulink Converter18/1 -> [Pdrop_hose_4]
  [P_T_big] -> Subtract1/1
  [P_A_big] -> Subtract1/2
  [Q_T_big] -> Scope16/1  "Q_T_big"
  [Q_P_big] -> Scope16/2  "Q_P_big"
  [Pdrop_hose_1] -> Product1/1
  [Q_A_big] -> Product1/2
  Product1/1 -> Integrator5/1
  Integrator5/1 -> Display6/1, Add5/1
  [Pdrop_hose_2] -> Product4/1
  [Q_P_small] -> Product4/2
  Product4/1 -> Integrator6/1
  Integrator6/1 -> Display7/1, Add5/2
  [Pdrop_hose_3] -> Product5/1
  [Q_T_small] -> Product5/2
  Product5/1 -> Integrator8/1
  Integrator8/1 -> Display8/1, Add5/3
  [Pdrop_hose_4] -> Product6/1
  [Qout] -> Product6/2
  Product6/1 -> Integrator9/1
  Integrator9/1 -> Add5/4, Display9/1
  Add5/1 -> Scope37/1, Display10/1, [Hose_loss]
  [Throttling_1] -> Add6/1
  [Throttling_2] -> Add6/2
  Add6/1 -> Throttling Total/1, [Throttling]
  [P1] -> To Workspace3/1, Scope/1  "P1"
  [Pdes] -> Scope/2  "Pdes"
  PS-Simulink Converter19/1 -> Scope17/1, [omega_dot]
  [omega] -> Product7/2
  [omega_dot] -> Product7/1
  Product7/1 -> Gain6/1
  Gain6/1 -> To Workspace7/1, Integrator16/1
  Integrator16/1 -> Mechanical Energy/1
  Subtract2/1 -> Stored/1, Scope21/1, To Workspace/1
  [omega] -> Scope5/4
  PS-Simulink Converter20/1 -> Goto30/1, Scope22/1
  PS-Simulink Converter21/1 -> [T_elec_2], To Workspace4/1, Scope23/2
  PS-Simulink Converter22/1 -> Scope24/1
  Gain/1 -> DC Current Controller/1, Scope25/1  "Desired"
  From46/1 -> DC Current Controller/2, Scope25/2  "Actual"
  DC Current Controller/1 -> Scope24/2, Simulink-PS Converter2/1
  Constant7/1 -> DC Current Controller/3
  Constant8/1 -> DC Current Controller/4
  From54/1 -> Gain7/1
  Gain7/1 -> Simulink-PS Converter3/1  "Desired"
  Integrator12/1 -> Regen1/1, To Workspace12/1, [Regen_Elec], Scope29/1  "Regen"
  Product9/1 -> Integrator12/1, To Workspace13/1, Scope28/1
  Product12/1 -> Integrator13/1
  From62/1 -> Product11/2
  Constant9/1 -> Product11/1
  From63/1 -> Product12/2
  Product11/1 -> Product12/1
  PS-Simulink Converter23/1 -> Display11/1, [P_B_small]
  PS-Simulink Converter24/1 -> [P_A_small], Display12/1
  [P_P_small] -> MATLAB Function3/3(P_P_small)
  [Qout] -> MATLAB Function3/7(Qout)
  [P_A_small] -> MATLAB Function3/1(P_A_small)
  [S_small] -> MATLAB Function3/5(S_small)
  MATLAB Function3/1(Power_loss_2) -> Abs2/1
  Integrator14/1 -> Scope32/1, Throttling Loss Small Valve1/1, [Throttling_2]
  [P_B_small] -> MATLAB Function3/2(P_B_small)
  [P_T_small] -> MATLAB Function3/4(P_T_small)
  [Q_A_big] -> MATLAB Function3/6(Q_A_big)
  PS-Simulink Converter25/1 -> [delP_pump]
  PS-Simulink Converter26/1 -> [pump_flow]
  Gain4/1 -> Gain5/1
  [P_P_big] -> MATLAB Function4/1(P_H_rail)
  Add3/1 -> To Workspace10/1, Add1/1, Scope15/1
  Integrator2/1 -> Add3/2
  Square1/1 -> Gain4/1
  MATLAB Function4/2(Power_out_2) -> Integrator2/1
  Gain5/1 -> Add1/2, To Workspace9/1, Initial Kinetic Energy/1
  Integrator/1 -> Add3/1
  Gain2/1 -> Display13/1, To Workspace2/1, Add/5
  Gain1/1 -> Gain2/1
  MATLAB Function4/1(Power_out_1) -> Integrator/1
  [P_T_big] -> MATLAB Function4/2(P_M_rail)
  [omega] -> Square2/1
  Constant1/1 -> Square1/1
  [Work_Out] -> Add/4
  [Q_T_big] -> MATLAB Function4/4(Q_T_big)
  Square2/1 -> Gain1/1
  [Q_P_big] -> MATLAB Function4/3(Q_P_big)
  Add1/1 -> Scope8/2, To Workspace8/1, Subtract2/1, Energy In/1  "In"
  Add/1 -> Energy Out/1, Subtract2/2, Scope8/1  "Out"
  [T_elec] -> Simulink-PS Converter4/1
  [Hose_loss] -> Add7/1
  [Throttling] -> Add7/2
  Add7/1 -> Add8/2, Add/2, To Workspace14/1
  PS-Simulink Converter27/1 -> [T_hyd], Scope23/1
  [T_elec_2] -> Product2/1, To Workspace15/1
  [Regen_Elec] -> Add1/3
  [Pump_Losses] -> Add8/3, Add/3
  [EMF] -> Product9/1
  [Current_arm] -> Product9/2
  [elec_motor_losses] -> Add/1, Add8/1
  [Q_T_small] -> Scope41/1
  [Q_P_small] -> Scope41/2
  Abs2/1 -> Integrator14/1
  Integrator21/1 -> Display15/1, Scope39/1, To Workspace17/1, [elec_motor_losses]
  Product14/1 -> Subtract3/2  "Mechanical_2"
  [omega] -> Product14/2
  [T_elec_2] -> MATLAB Function6/1(T_elec_2)
  MATLAB Function6/3(I_elec) -> Scope18/1, [Current_arm]
  Abs1/1 -> Integrator21/1
  Integrator20/1 -> [Pump_Losses], To Workspace16/1, Display14/1, Scope38/1
  Abs/1 -> Integrator20/1
  Subtract4/1 -> Abs1/1
  MATLAB Function6/1(Elec_Power) -> Scope27/2, Subtract4/2
  [T_hyd] -> Product14/1
  [pump_flow] -> Product13/2
  Subtract3/1 -> Abs/1
  [omega] -> MATLAB Function6/2(omega)
  [T_elec_2] -> Product8/2
  Product8/1 -> Scope27/1, Subtract4/1  "Mechanical"
  Integrator15/1 -> [Pump_Hyd_Energy]  "Hyd"
  MATLAB Function6/2(V_elec) -> [EMF]
  Product13/1 -> Subtract3/1, Integrator15/1  "Hydraulic"
  [omega] -> Product8/1
  [delP_pump] -> Product13/1
  Gain8/1 -> Gain3/1
  Gain3/1 -> Integrator4/1
  Integrator4/1 -> Gain9/1
  Gain9/1 -> Scope26/1, Display16/1
  Add8/1 -> To Workspace20/1, Scope31/1
  [Q_P_small] -> MATLAB Function3/8(Q_P_small)
  [Q_T_small] -> MATLAB Function3/9(Q_T_small)
  MATLAB Function3/2(Power_loss_middle) -> Scope42/1
  [omega] -> Gain10/1
  Gain10/1 -> Product10/1
  [omega] -> Product10/2
  Product10/1 -> Integrator10/1
  Integrator10/1 -> [damping_losses]
  connections:
  Solver Configuration1/RConn1 -- PS Constant/RConn1 -- Pressure Source (IL)1/LConn2
  Reservoir (IL)5/LConn1 -- Isothermal Liquid Properties (IL)/RConn1 -- Pressure Source (IL)1/LConn1
  Mechanical Translational Reference2/LConn1 -- Double-Acting Actuator (IL)1/LConn1
  Mechanical Translational Reference3/LConn1 -- Double-Acting Actuator (IL)1/RConn2
  Reservoir (IL)7/LConn1 -- Double-Acting Actuator (IL)1/RConn3
  Flow Rate Sensor (IL)/RConn1 -- Double-Acting Actuator (IL)1/LConn2 -- Pressure Sensor (IL)2/LConn1
  PS-Simulink Converter3/LConn1 -- Pressure Sensor (IL)2/RConn1
  Pressure Sensor (IL)4/LConn1 -- 4-Way 2-Position Directional Valve (IL)/LConn2 -- Flow Rate Sensor (IL)2/LConn1
  Fixed-Displacement Motor (IL)/RConn2 -- Rotational Damper/RConn1 -- Ideal Torque Source/RConn2 -- Ideal Rotational Motion Sensor1/RConn1 -- Mechanical Rotational Reference2/LConn1
  Ideal Rotational Motion Sensor1/LConn1 -- Hydraulic Motor Inertia/LConn1 -- Ideal Torque Sensor1/RConn1 -- Ideal Torque Sensor/RConn1
  PS-Simulink Converter5/LConn1 -- Liquid Properties Sensor (IL)/RConn2
  PS-Simulink Converter6/LConn1 -- Liquid Properties Sensor (IL)/RConn1
  Flow Rate Sensor (IL)/RConn2 -- PS-Simulink Converter/LConn1
  Pipe (IL)5/LConn1 -- Pressure Sensor (IL)9/RConn1 -- Flow Rate Sensor (IL)/LConn1
  Simulink-PS Converter1/RConn1 -- 4-Way 3-Position Directional Valve (IL)/LConn1
  Liquid Properties Sensor (IL)/LConn1 -- Pressure Source (IL)1/RConn1 -- Flow Rate Sensor (IL)1/LConn1
  Pressure Sensor (IL)3/LConn1 -- 4-Way 2-Position Directional Valve (IL)/RConn1 -- Flow Rate Sensor (IL)1/RConn1
  Flow Rate Sensor (IL)2/RConn1 -- Pressure Sensor (IL)6/LConn1 -- Pipe (IL)2/LConn1
  PS-Simulink Converter7/LConn1 -- Pressure Sensor (IL)3/RConn1
  PS-Simulink Converter8/LConn1 -- Pressure Sensor (IL)4/RConn1
  PS-Simulink Converter9/LConn1 -- Flow Rate Sensor (IL)2/RConn2
  Flow Rate Sensor (IL)3/LConn1 -- Pressure Sensor (IL)1/LConn1 -- 4-Way 3-Position Directional Valve (IL)/RConn1
  Flow Rate Sensor (IL)3/RConn1 -- Pressure Sensor (IL)7/LConn1 -- Pipe (IL)4/LConn1
  Flow Rate Sensor (IL)4/LConn1 -- Pressure Sensor (IL)5/LConn1 -- 4-Way 3-Position Directional Valve (IL)/RConn2
  Flow Rate Sensor (IL)4/RConn1 -- Pressure Sensor (IL)8/LConn1 -- Pipe (IL)3/LConn1
  PS-Simulink Converter2/LConn1 -- Pressure Sensor (IL)5/RConn1
  PS-Simulink Converter10/LConn1 -- Pressure Sensor (IL)1/RConn1
  PS-Simulink Converter11/LConn1 -- Flow Rate Sensor (IL)3/RConn2
  PS-Simulink Converter12/LConn1 -- Flow Rate Sensor (IL)4/RConn2
  PS Constant1/RConn1 -- Pressure Source (IL)2/LConn2
  Reservoir (IL)1/LConn1 -- Pressure Source (IL)2/LConn1
  Flow Rate Sensor (IL)5/LConn1 -- Pressure Sensor (IL)/LConn1 -- Pressure Source (IL)2/RConn1
  Flow Rate Sensor (IL)5/RConn1 -- 4-Way 2-Position Directional Valve (IL)/RConn2
  PS-Simulink Converter13/LConn1 -- Flow Rate Sensor (IL)5/RConn2
  PS-Simulink Converter4/LConn1 -- Flow Rate Sensor (IL)1/RConn2
  Pressure Sensor (IL)6/RConn1 -- Flow Rate Sensor (IL)7/LConn1 -- Pipe (IL)2/RConn1
  Pipe (IL)3/RConn1 -- Fixed-Displacement Motor (IL)/RConn3 -- Pressure Sensor (IL)8/RConn1 -- Pressure Sensor (IL)12/RConn1
  Pipe (IL)4/RConn1 -- Flow Rate Sensor (IL)6/LConn1 -- Pressure Sensor (IL)7/RConn1
  4-Way 3-Position Directional Valve (IL)/LConn3 -- Pressure Sensor (IL)9/LConn1 -- Pipe (IL)5/RConn1 -- Pressure Sensor (IL)10/LConn1
  Simulink-PS Converter/RConn1 -- 4-Way 2-Position Directional Valve (IL)/LConn1
  4-Way 2-Position Directional Valve (IL)/LConn3 -- Reservoir (IL)8/LConn1
  PS-Simulink Converter14/LConn1 -- Pressure Sensor (IL)/RConn1
  PS-Simulink Converter15/LConn1 -- Pressure Sensor (IL)6/RConn2
  PS-Simulink Converter16/LConn1 -- Pressure Sensor (IL)7/RConn2
  PS-Simulink Converter17/LConn1 -- Pressure Sensor (IL)8/RConn2
  PS-Simulink Converter18/LConn1 -- Pressure Sensor (IL)9/RConn2
  Ideal Rotational Motion Sensor1/RConn3 -- PS-Simulink Converter1/LConn1
  PS-Simulink Converter19/LConn1 -- Ideal Rotational Motion Sensor1/RConn2
  Electrical Reference/LConn1 -- Voltage Sensor/RConn2 -- DC Motor/RConn1 -- Controlled Voltage Source/RConn2
  PS-Simulink Converter20/LConn1 -- Current Sensor/RConn1
  Voltage Sensor/LConn1 -- Current Sensor/RConn2 -- DC Motor/LConn1
  PS-Simulink Converter21/LConn1 -- Ideal Torque Sensor/RConn2
  PS-Simulink Converter22/LConn1 -- Voltage Sensor/RConn1
  Simulink-PS Converter2/RConn1 -- Controlled Voltage Source/RConn1
  Simulink-PS Converter3/RConn1 -- Controlled Current Source/RConn1
  Controlled Voltage Source/LConn1 -- Current Sensor/LConn1
  PS-Simulink Converter23/LConn1 -- Pressure Sensor (IL)10/RConn1
  PS-Simulink Converter24/LConn1 -- Pressure Sensor (IL)11/RConn1
  PS-Simulink Converter25/LConn1 -- Pressure Sensor (IL)12/RConn2
  Flow Rate Sensor (IL)6/RConn1 -- Fixed-Displacement Motor (IL)/LConn1 -- Pressure Sensor (IL)12/LConn1
  PS-Simulink Converter26/LConn1 -- Flow Rate Sensor (IL)6/RConn2
  Simulink-PS Converter4/RConn1 -- Ideal Torque Source/RConn1
  Pressure Sensor (IL)11/LConn1 -- Flow Rate Sensor (IL)7/RConn1 -- 4-Way 3-Position Directional Valve (IL)/LConn2
  Ideal Torque Sensor1/LConn1 -- Rotational Damper/LConn1 -- Fixed-Displacement Motor (IL)/RConn1
  PS-Simulink Converter27/LConn1 -- Ideal Torque Sensor1/RConn2
  Ideal Torque Source/LConn1 -- Ideal Torque Sensor/LConn1

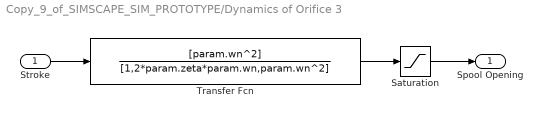
== system Copy_9_of_SIMSCAPE_SIM_PROTOTYPE/Dynamics of Orifice 3 ==
  Stroke : Inport
  Saturation : Saturate  UpperLimit=param.stroke  LowerLimit=0
  Transfer Fcn : TransferFcn  Numerator=[param.wn^2]  Denominator=[1,2*param.zeta*param.wn,param.wn^2]
  Spool Opening : Outport
  wires:
  Transfer Fcn/1 -> Saturation/1
  Saturation/1 -> Spool Opening/1
  Stroke/1 -> Transfer Fcn/1
